simulink model "LaunchControlAttempt2"  (R2024b)
settings: Solver=ode45  StartTime=0.0  StopTime=5  MaxStep=0.0002  RelTol=1e-3
undefined symbols (not defined in the file or in its folder): DTParameters, g, lr, m, TireParameters, VParameters
libraries: slpidlib x1, autolibshared x1
settings Model: Creator=nhola  LastModifiedBy=2017w
settings DataIOCC: ExternalInput=[Tire, Parameter]
settings DebuggingCC: AlgebraicLoopMsg=none  UnderSpecifiedDimensionMsg=warning

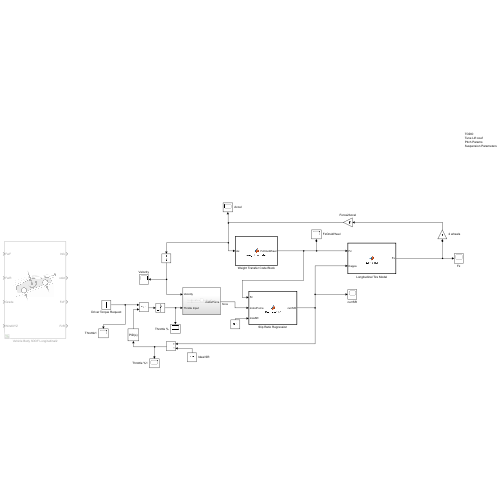
[thumbnail: Simulink's stored preview of the top-level diagram]
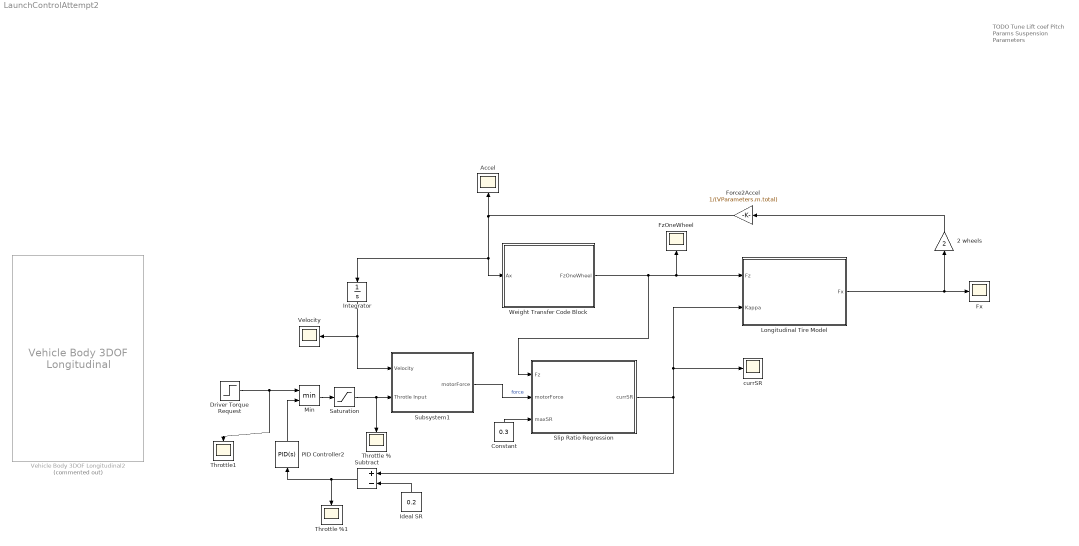
== system LaunchControlAttempt2 ==
  note: TODO
      | Tune Lift coef
      | Pitch Params
      | Suspension Parameters
  2 wheels : Gain  Gain=2
  Accel : Scope
  Constant : Constant  Value=0.3
  Driver Torque Request : Step  Time=0.05  After=100  SampleTime=0
  Force2Accel : Gain  Gain=1/(VParameters.m.total)
  Fx : Scope
  FzOneWheel : Scope
  Ideal SR : Constant  Value=0.2
  Integrator : Integrator
  Longitudinal Tire Model : MATLAB Function  TreatAsAtomicUnit=on
  Min : MinMax  Inputs=2
  PID Controller2 : slpidlib/PID Controller  Controller=PID  Form=Parallel  TimeDomain=Continuous-time  UseExternalTs=off  SampleTime=-1  IntegratorMethod=Forward Euler  FilterMethod=Forward Euler  ControllerParametersSource=internal  P=1000  I=100  UseKiTs=off  D=20  UseExternalDerivativeSource=off  N=0  UseFilter=on  TunerSelectOption=Transfer Function Based (PID Tuner App)  InitialConditionSource=internal  InitialConditionForIntegrator=0  InitialConditionForFilter=0  DifferentiatorICPrevScaledInput=0  ExternalReset=none  TrackingMode=off  Kt=1  LimitOutput=off  SatLimitsSource=internal  UpperSaturationLimit=inf  LowerSaturationLimit=-inf  LinearizeAsGain=on  AntiWindupMode=none  Kb=1  LimitIntegrator=off  UpperIntegratorSaturationLimit=inf  LowerIntegratorSaturationLimit=-inf  POutMin=[]  POutMax=[]  IOutMin=[]  IOutMax=[]  DOutMin=[]  DOutMax=[]  NOutMin=[]  NOutMax=[]  SumOutMin=[]  SumOutMax=[]  SaturationOutMin=[]  SaturationOutMax=[]  PParamMin=[]  PParamMax=[]  IParamMin=[]  IParamMax=[]  DParamMin=[]  DParamMax=[]  NParamMin=[]  NParamMax=[]  KbParamMin=[]  KbParamMax=[]  KtParamMin=[]  KtParamMax=[]  KbOutMin=[]  KbOutMax=[]  KtOutMin=[]  KtOutMax=[]  IntegratorOutMin=[]  IntegratorOutMax=[]  FilterOutMin=[]  FilterOutMax=[]  SumI1OutMin=[]  SumI1OutMax=[]  SumI2OutMin=[]  SumI2OutMax=[]  SumI3OutMin=[]  SumI3OutMax=[]  SumI4OutMin=[]  SumI4OutMax=[]  SumDOutMin=[]  SumDOutMax=[]  DifferentiatorOutMin=[]  DifferentiatorOutMax=[]  FilterDiffOutCoefMin=[]  FilterDiffOutCoefMax=[]  ReciprocalOutMin=[]  ReciprocalOutMax=[]  SumDenOutMin=[]  SumDenOutMax=[]  SumNumOutMin=[]  SumNumOutMax=[]  DivideOutMin=[]  DivideOutMax=[]  UdiffTsProdOutMin=[]  UdiffTsProdOutMax=[]  NTsProdOutMin=[]  NTsProdOutMax=[]  UintegralTsProdOutMin=[]  UintegralTsProdOutMax=[]  UngainTsProdOutMin=[]  UngainTsProdOutMax=[]  ClampingZeroOutDataTypeStr=Inherit: Inherit via back propagation  ClampingZeroOutMin=[]  ClampingZeroOutMax=[]  FilterDenConstantOutDataTypeStr=Inherit: Inherit via back propagation  FilterDenConstantOutMin=[]  FilterDenConstantOutMax=[]  PCopyOutDataTypeStr=Inherit: Inherit via back propagation  PCopyOutMin=[]  PCopyOutMax=[]  NCopyOutDataTypeStr=Inherit: Inherit via back propagation  NCopyOutMin=[]  NCopyOutMax=[]  IntegratorContinuousStateAttributes=''  IntegratorStateMustResolveToSignalObject=off  IntegratorRTWStateStorageClass=Auto  FilterContinuousStateAttributes=''  FilterStateMustResolveToSignalObject=off  FilterRTWStateStorageClass=Auto  ParallelPVariant=InternalParameters  IdealPVariant=Disabled  IVariant=InternalParameters  DVariant=InternalParameters  IntegratorVariant=Continuous  SatVariant=Disabled  AWVariant=Passthrough  PCopyVariant=Disabled  TRVariant=Disabled  FdbkBlocksVariant=Forward  IdealPFdbkVariant=Disabled  SatFdbkVariant=Disabled  DerivativeFilterVariant=ContFilter  NVariant=InternalParameters  NCopyVariant=Disabled  FilterICVariant=InternalICsFilter  IntegratorICVariant=InternalICs  ExternalResetVariant=Disabled  TRSumVariant=Passthrough  SumFdbkVariant=Disabled  SumVariant=Sum_PID  TsampFilterVariant=InternalTs  TsampNgainVariant=Passthrough  TsampIntegralVariant=Disabled_SignalSpec  ExternalSaturationOutDataTypeStr=Inherit: Same as second input  DerivativeSourceVariant=ErrorSignal  PreIntVariant=InternalPreInt
  Saturation : Saturate  UpperLimit=100  LowerLimit=0
  Slip Ratio Regression : MATLAB Function  TreatAsAtomicUnit=on
  Subsystem1 : Subsystem
  Subtract : Sum  Inputs=+-
  Throttle % : Scope
  Throttle %1 : Scope
  Throttle1 : Scope
  Vehicle Body 3DOF Longitudinal2 : autolibshared/Vehicle Body 3DOF Longitudinal  Commented=on  VariantControl=SL  groundType=Grade angle  aMode=2  extFMode=off  extMMode=off  extTamb=off  NF=2  NR=2  m=m.total  a=lf  b=lr  h=hCG  Cd=Cd  Af=A_ref  x_o=0  xdot_o=0  Cl=-0.5  z_o=0  zdot_o=0  Iyy=1500  Cpm=.1  theta_o=0  q_o=0  FskF=[-50, -1, 0, 2, 3, 52].*1.5e4  dzsF=[-5e-3, -1e-4, 0, .2, .2001, .2051]  FsbF=[-10000 -100 -10 0 10 100 10000]  dzdotsF=[-10 -1 -.1 0 .1 1 10]  FskR=[-50, -1, 0, 2, 3, 52].*1e4  dzsR=[-5e-3, -1e-4, 0, .2, .2001, .2051]  FsbR=[-10000 -100 -10 0 10 100 10000]  dzdotsR=[-10 -1 -.1 0 .1 1 10]  Pabs=101325  T=273  g=g  blkID=0
      settings: LibrarySourceBlock=vehdynlibeom/Vehicle Body 3DOF Longitudinal
  Velocity : Scope
  Weight Transfer Code Block : MATLAB Function  TreatAsAtomicUnit=on
  currSR : Scope
  wires:
  Longitudinal Tire Model/1(Fx) -> Fx/1, 2 wheels/1
  2 wheels/1 -> Force2Accel/1
  Driver Torque Request/1 -> Throttle1/1, Min/1
  Subtract/1 -> PID Controller2/1, Throttle %1/1
  Ideal SR/1 -> Subtract/2
  Min/1 -> Saturation/1
  Subsystem1/1(motorForce) -> Slip Ratio Regression/2(motorForce)  "force"
  Slip Ratio Regression/1(currSR) -> Longitudinal Tire Model/2(Kappa), currSR/1, Subtract/1
  Integrator/1 -> Velocity/1, Subsystem1/1(Velocity)
  Constant/1 -> Slip Ratio Regression/3(maxSR)
  Weight Transfer Code Block/1(FzOneWheel) -> Slip Ratio Regression/1(Fz), FzOneWheel/1, Longitudinal Tire Model/1(Fz)
  Force2Accel/1 -> Accel/1, Integrator/1, Weight Transfer Code Block/1(Ax)
  Saturation/1 -> Subsystem1/2(Throtle Input), Throttle %/1
  PID Controller2/1 -> Min/2

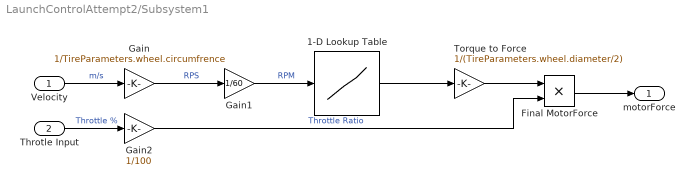
== system LaunchControlAttempt2/Subsystem1 ==
  Velocity : Inport
  Throtle Input : Inport  Port=2
  1-D Lookup Table : Lookup_n-D  NumberOfTableDimensions=1  BreakpointsForDimension1=DTParameters.torque_vs_RPM_breakpoints  Table=DTParameters.torque_vs_RPM_table  ExtrapMethod=Clip  UseLastTableValue=on  InternalRulePriority=Speed  RndMeth=Simplest
  Final MotorForce : Product
  Gain : Gain  Gain=1/TireParameters.wheel.circumfrence
  Gain1 : Gain  Gain=1/60
  Gain2 : Gain  Gain=1/100
  Torque to Force : Gain  Gain=1/(TireParameters.wheel.diameter/2)
  motorForce : Outport
  wires:
  Velocity/1 -> Gain/1  "m/s"
  Gain/1 -> Gain1/1  "RPS"
  Gain1/1 -> 1-D Lookup Table/1  "RPM"
  1-D Lookup Table/1 -> Torque to Force/1
  Throtle Input/1 -> Gain2/1  "Throttle %"
  Gain2/1 -> Final MotorForce/2  "Throttle Ratio"
  Torque to Force/1 -> Final MotorForce/1
  Final MotorForce/1 -> motorForce/1

== matlab function LaunchControlAttempt2/Weight Transfer Code Block ==
  data: Ax input; FzOneWheel output; VParameters parameter
function FzOneWheel = weightTransfer(Ax, VParameters)
    
    deltaFz = Ax .* VParameters.hCG .* VParameters.m.total ./ VParameters.wheelBase ;
    deltaFz = deltaFz ./2; % Weight Transfer in each wheel in the back
    FzOneWheel = VParameters.m.total .* 9.81 .* (VParameters.lf ./ VParameters.wheelBase) ./2 + deltaFz;

end

== matlab function LaunchControlAttempt2/Longitudinal Tire Model ==
  data: Fz input; Kappa input; Fx output; TireParameters parameter
function Fx = LongTM(Fz,Kappa, TireParameters)
    
    Pi = 70;
    Inc = 0;
    
    dFz = (Fz - TireParameters.Pacejka.Fzo) ./ TireParameters.Pacejka.Fzo;
    dPi = (Pi - TireParameters.Pacejka.Pio) ./ TireParameters.Pacejka.Pio;
    
    Cx = TireParameters.Pacejka.p.C.x(1) .* TireParameters.Pacejka.L.C.x;
    
    Dx = (TireParameters.Pacejka.p.D.x(1) + TireParameters.Pacejka.p.D.x(2).*dFz) .* ...
         (1 + TireParameters.Pacejka.p.P.x(3).*dPi + TireParameters.Pacejka.p.P.x(4).*dPi.^2) .* ...
         (1 - TireParameters.Pacejka.p.D.x(3).*Inc.^2).*Fz .* TireParameters.Pacejka.L.mu.x;
    
    Ex = ( TireParameters.Pacejka.p.E.x(1) + TireParameters.Pacejka.p.E.x(2).*dFz ...
        + TireParameters.Pacejka.p.E.x(3).*dFz.^2 ) .* ( 1 - TireParameters.Pacejka.p.E.x(4).*sign(Kappa) ) .* ...
        TireParameters.Pacejka.L.E.x;
    
    Kxk = Fz.*(TireParameters.Pacejka.p.K.x(1) + TireParameters.Pacejka.p.K.x(2).*dFz ) .* ...
        exp( TireParameters.Pacejka.p.K.x(3) .* dFz ) .* ...
        (1 + TireParameters.Pacejka.p.P.x(1).*dPi + TireParameters.Pacejka.p.P.x(2).*dPi.^2) .* ...
        TireParameters.Pacejka.L.K.x.k;
    
    Bx = Kxk ./ ( Cx.*Dx );
    
    Vx = Fz.*(TireParameters.Pacejka.p.V.x(1) + TireParameters.Pacejka.p.V.x(2).*dFz ) .* ...
        TireParameters.Pacejka.L.V.x;
    
    Hx = (TireParameters.Pacejka.p.H.x(1) + TireParameters.Pacejka.p.H.x(2).*dFz) .* ...
        TireParameters.Pacejka.L.H.x;
    
    Fx = Dx .* sin( Cx .* atan( (1-Ex) .* Bx.*(Kappa + Hx) + ...
        Ex.*atan( Bx.*(Kappa + Hx) ) ) ) + Vx;

end

== matlab function LaunchControlAttempt2/Slip Ratio Regression ==
  data: Fz input; motorForce input; currSR output; maxSR input; TireParameters parameter
function currSR = RegressSR(Fz, motorForce, maxSR, TireParameters)
    currSR = 0.0; % Assign variable Type Double
    
    % disp(Fz)
    % disp(motorForce)
    % disp('-------------------------------------------------')

    coder.extrinsic('regressSRFunction');
    currSR = regressSRFunction(Fz, motorForce, maxSR, TireParameters);

    if currSR < 9.5e-5
        currSR = 0;
    end
end



function Fx = LongTM(Fz,Kappa, TireParameters)
    
    Pi = 70;
    Inc = 0;
    
    dFz = (Fz - TireParameters.Pacejka.Fzo) ./ TireParameters.Pacejka.Fzo;
    dPi = (Pi - TireParameters.Pacejka.Pio) ./ TireParameters.Pacejka.Pio;
    
    Cx = TireParameters.Pacejka.p.C.x(1) .* TireParameters.Pacejka.L.C.x;
    
    Dx = (TireParameters.Pacejka.p.D.x(1) + TireParameters.Pacejka.p.D.x(2).*dFz) .* ...
         (1 + TireParameters.Pacejka.p.P.x(3).*dPi + TireParameters.Pacejka.p.P.x(4).*dPi.^2) .* ...
         (1 - TireParameters.Pacejka.p.D.x(3).*Inc.^2).*Fz .* TireParameters.Pacejka.L.mu.x;
    
    Ex = ( TireParameters.Pacejka.p.E.x(1) + TireParameters.Pacejka.p.E.x(2).*dFz ...
        + TireParameters.Pacejka.p.E.x(3).*dFz.^2 ) .* ( 1 - TireParameters.Pacejka.p.E.x(4).*sign(Kappa) ) .* ...
        TireParameters.Pacejka.L.E.x;
    
    Kxk = Fz.*(TireParameters.Pacejka.p.K.x(1) + TireParameters.Pacejka.p.K.x(2).*dFz ) .* ...
        exp( TireParameters.Pacejka.p.K.x(3) .* dFz ) .* ...
        (1 + TireParameters.Pacejka.p.P.x(1).*dPi + TireParameters.Pacejka.p.P.x(2).*dPi.^2) .* ...
        TireParameters.Pacejka.L.K.x.k;
    
    Bx = Kxk ./ ( Cx.*Dx );
    
    Vx = Fz.*(TireParameters.Pacejka.p.V.x(1) + TireParameters.Pacejka.p.V.x(2).*dFz ) .* ...
        TireParameters.Pacejka.L.V.x;
    
    Hx = (TireParameters.Pacejka.p.H.x(1) + TireParameters.Pacejka.p.H.x(2).*dFz) .* ...
        TireParameters.Pacejka.L.H.x;
    
    Fx = Dx .* sin( Cx .* atan( (1-Ex) .* Bx.*(Kappa + Hx) + ...
        Ex.*atan( Bx.*(Kappa + Hx) ) ) ) + Vx;

end
